simulink model "ddmr_for_mstc2003"  (R2022a)
settings: Solver=ode45  StartTime=0.0  StopTime=15  MaxStep=.1  MinStep=.001  RelTol=1e-3  EnableMultiTasking=on
libraries: dspsigattribs x28, matrix_library x6, dspinverses x3
settings Model: Creator=Orsted  LastModifiedBy=Orsted
settings SolverCC: InitialStep=.001
settings DataIOCC: LimitDataPoints=on  MaxDataPoints=10000  SaveFormat=Array  SignalLoggingSaveFormat=ModelDataLogs  ReturnWorkspaceOutputs=off  SignalLoggingName=sigsOut
settings OptimizationCC: BooleanDataType=off
settings DebuggingCC: SaveWithParameterizedLinksMsg=none  UnderspecifiedInitializationDetection=Classic  MergeDetectMultiDrivingBlocksExec=none  SignalResolutionControl=TryResolveAllWithWarning  MultiTaskDSMMsg=warning  MultiTaskCondExecSysMsg=none  UnconnectedInputMsg=warning  UnconnectedOutputMsg=warning  UnconnectedLineMsg=warning
settings HardwareCC: ProdBitPerPointer=32  ProdBitPerSizeT=32  ProdBitPerPtrDiffT=32  ProdLargestAtomicFloat=None  ProdIntDivRoundTo=Undefined  ProdEndianess=Unspecified  ProdWordSize=32  ProdHWDeviceType=32-bit Generic  TargetUnknown=on
settings ModelReferenceCC: PropagateSignalLabelsOutOfModel=off
settings GRTTargetCC: CombineOutputUpdateFcns=off  GRTInterface=on
settings ConfigComp: CovMetricSettings=dw  CovSaveCumulativeToWorkspaceVar=on  CovSaveSingleToWorkspaceVar=on

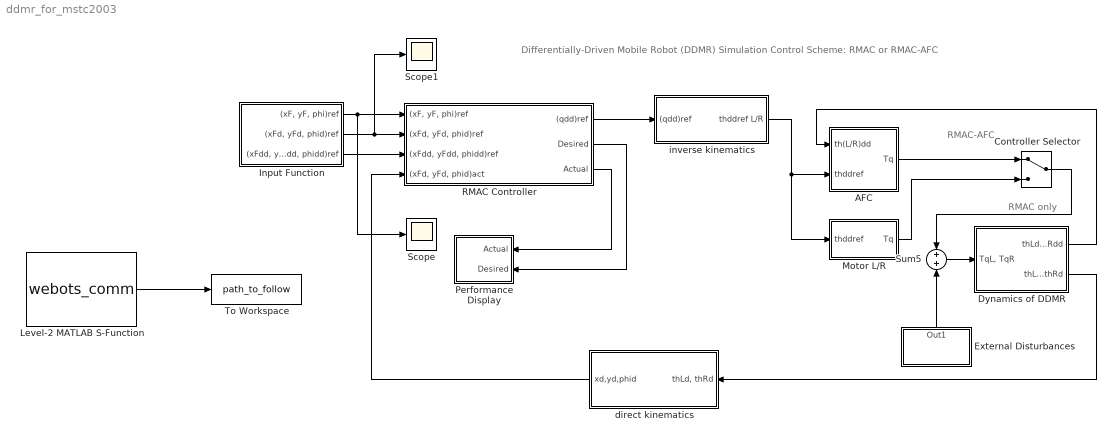
== system ddmr_for_mstc2003 ==
  note: Differentially-Driven Mobile Robot (DDMR) Simulation
      | Control Scheme: RMAC or RMAC-AFC
  note: RMAC-AFC
  note: RMAC only
  AFC : Subsystem  mask{IN=2.4, Ktn=.263}
      mask prompts: IN "Crude's Value (IN)"; Ktn "Motor Constant (Ktn)"
  Controller Selector : ManualSwitch
  Dynamics of DDMR : Subsystem  mask{phi=pi/2, d=.3, r=.11, mw=1, mc=40, b=.4, Ic=11.525, Im=.05, Iw=0.05}
      mask prompts: phi "Vehicle initial orientation (phi)"; d "Distance between Po to Pc (d)"; r "Radius of Wheels (r)"; mw "Mass of wheel (mw)"; mc "Mass of platform (mc)"; b "(1/2)Width of vehicle (b)"; Ic "Inertia of platform about vertical axis (Ic)"; Im "Inertia of wheel about wheel diameter (Im)"; Iw "Inertia of wheel about wheel axis (Iw)"
  External Disturbances : Subsystem  mask{Qtype=[5;6], Qc=[5;-5], Qpa=2, Qpf=1, Qsa=5, Qsf=5}
      mask prompts: Qtype "Disturbance Type: [1;2]Qconstant  [3;4]Qpulse  [5;6]Qsine"; Qc "Magnitude of Q-Constant (Qc)"; Qpa "Amplitude of Q-Pulse (Qpa)"; Qpf "Freq of Q-Pulse (Qpf)"; Qsa "Amplitude of Q-Sine (Qsa)"; Qsf "Freq of Q-Sine (Qsa)"
  Input Function : Subsystem  mask{phiref=pi/2, InSet=4, Vcut=.4, rinput=10}
      mask prompts: phiref "Vehicle Initial orientation (phiref)"; InSet "Input [ <1>Line-1 <2>Line-2 <3>Line-3 <4>Curve ]"; Vcut "Velocity of Running (Curve only)"; rinput "Radius of Curve"
  Level-2 MATLAB S-Function : M-S-Function  FunctionName=webots_comm
  Motor L/R : Subsystem
  Performance Display : Subsystem
  RMAC Controller : Subsystem  mask{qinit=[7;0;pi/2], Kp=[350;350;.005], Kd=[320;320;.0015]}
      mask prompts: qinit "Vehicle initial position (xF, yF, phi) > (qinit)"; Kp "Proportional Constant (Kp)"; Kd "Differential Constant (Kd)"
  Scope : Scope
  Scope1 : Scope
  Sum5 : Sum  InputSameDT=on  SaturateOnIntegerOverflow=on  OutDataTypeStr=Inherit: Same as first input
  To Workspace : ToWorkspace  VariableName=path_to_follow  SaveFormat=Structure With Time  SampleTime=-1
  direct kinematics : Subsystem  mask{phi=pi/2, b=0.4, r=0.11, lG=.3}
      mask prompts: phi "Vehicle initial orientation (phi)"; b "(1/2)Width of Body, b (m)"; r "Radius of wheels, r (m)"; lG "Distance between WG to WF (lG)"
  inverse kinematics : Subsystem  mask{phi=pi/2, b=0.4, r=0.11, lG=.3}
      mask prompts: phi "Vehicle initial orientation (phi)"; b "(1/2)Width of Body, b (m)"; r "Radius of wheels, r (m)"; lG "Distance between WG to WF (lG)"
  wires:
  Input Function/2("(xFd, yFd, phid)ref") -> Scope1/1, RMAC Controller/2("(xFd, yFd, phid)ref")
  RMAC Controller/1((qdd)ref) -> inverse kinematics/1((qdd)ref)
  Dynamics of DDMR/2("thLd, thRd") -> direct kinematics/1("thLd, thRd")
  Sum5/1 -> Dynamics of DDMR/1("TqL, TqR")
  Input Function/1("(xF, yF, phi)ref") -> Scope/1, RMAC Controller/1("(xF, yF, phi)ref")
  direct kinematics/1(xd,yd,phid) -> RMAC Controller/4("(xFd, yFd, phid)act")
  Input Function/3("(xFdd, yFdd, phidd)ref") -> RMAC Controller/3("(xFdd, yFdd, phidd)ref")
  External Disturbances/1(Out1) -> Sum5/2
  RMAC Controller/3(Actual) -> Performance Display/1(Actual)
  RMAC Controller/2(Desired) -> Performance Display/2(Desired)
  Dynamics of DDMR/1("thLdd, thRdd") -> AFC/1(th(L/R)dd)
  inverse kinematics/1(thddref L/R) -> AFC/2(thddref), Motor L/R/1(thddref)
  AFC/1(Tq) -> Controller Selector/1
  Controller Selector/1 -> Sum5/1
  Motor L/R/1(Tq) -> Controller Selector/2
  Level-2 MATLAB S-Function/1 -> To Workspace/1

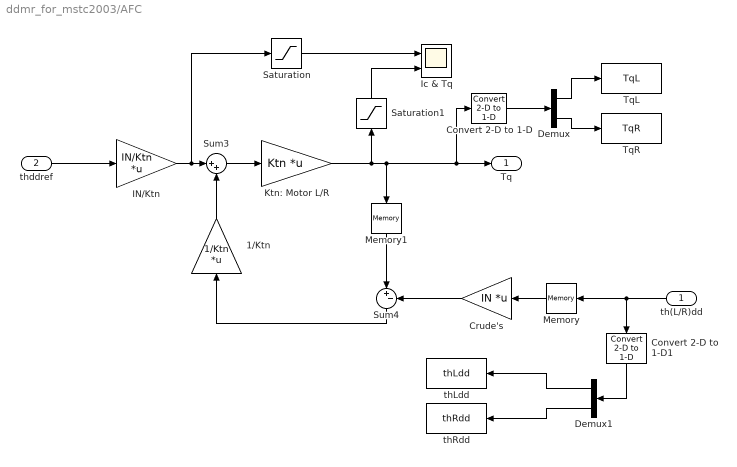
== system ddmr_for_mstc2003/AFC ==
  th(L/R)dd : Inport
  thddref : Inport  Port=2
  1/Ktn : Gain  Gain=1/Ktn  Multiplication=Matrix(K*u)  SaturateOnIntegerOverflow=on  OutDataTypeStr=Inherit: Same as input  ParamDataTypeStr=Inherit: Same as input
  Convert 2-D to 1-D : dspsigattribs/Convert 2-D to 1-D
      settings: SourceProductBaseCode=DS
  Convert 2-D to 1-D1 : dspsigattribs/Convert 2-D to 1-D
      settings: SourceProductBaseCode=DS
  Crude's : Gain  Gain=IN  Multiplication=Matrix(K*u)  SaturateOnIntegerOverflow=on  OutDataTypeStr=Inherit: Same as input  ParamDataTypeStr=Inherit: Same as input
  Demux : Demux  Outputs=2
      settings: DisplayOption=none
  Demux1 : Demux  Outputs=2
      settings: DisplayOption=none
  IN/Ktn : Gain  Gain=IN/Ktn  Multiplication=Matrix(K*u)  SaturateOnIntegerOverflow=on  OutDataTypeStr=Inherit: Same as input  ParamDataTypeStr=Inherit: Same as input
  Ic & Tq : Scope  NumInputPorts=2
  Ktn: Motor L/R : Gain  Gain=Ktn  Multiplication=Matrix(K*u)  SaturateOnIntegerOverflow=on  OutDataTypeStr=Inherit: Same as input  ParamDataTypeStr=Inherit: Same as input
  Memory : Memory
  Memory1 : Memory
  Saturation : Saturate  UpperLimit=30  LowerLimit=-30
  Saturation1 : Saturate  UpperLimit=30  LowerLimit=-30
  Sum3 : Sum  Inputs=|++  InputSameDT=on  SaturateOnIntegerOverflow=on  OutDataTypeStr=Inherit: Same as first input
  Sum4 : Sum  Inputs=|+-  InputSameDT=on  SaturateOnIntegerOverflow=on  OutDataTypeStr=Inherit: Same as first input
  TqL : ToWorkspace  VariableName=TqL  SampleTime=-1
  TqR : ToWorkspace  VariableName=TqR  SampleTime=-1
  thLdd : ToWorkspace  VariableName=thLdd  SampleTime=-1
  thRdd : ToWorkspace  VariableName=thRdd  SampleTime=-1
  Tq : Outport
  wires:
  Sum3/1 -> Ktn: Motor L/R/1
  IN/Ktn/1 -> Sum3/1, Saturation/1
  Crude's/1 -> Sum4/2
  Sum4/1 -> 1/Ktn/1
  1/Ktn/1 -> Sum3/2
  thddref/1 -> IN/Ktn/1
  th(L/R)dd/1 -> Memory/1, Convert 2-D to 1-D1/1
  Ktn: Motor L/R/1 -> Memory1/1, Tq/1, Convert 2-D to 1-D/1, Saturation1/1
  Saturation/1 -> Ic & Tq/1
  Saturation1/1 -> Ic & Tq/2
  Memory/1 -> Crude's/1
  Memory1/1 -> Sum4/1
  Demux/1 -> TqL/1
  Demux/2 -> TqR/1
  Convert 2-D to 1-D/1 -> Demux/1
  Demux1/1 -> thLdd/1
  Demux1/2 -> thRdd/1
  Convert 2-D to 1-D1/1 -> Demux1/1

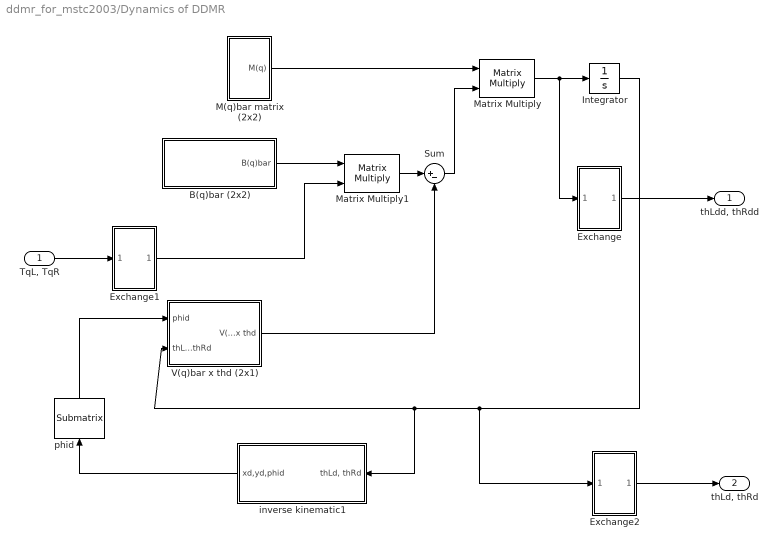
== system ddmr_for_mstc2003/Dynamics of DDMR ==
  "TqL, TqR" : Inport
  B(q)bar (2x2) : Subsystem
  Exchange : Subsystem
  Exchange1 : Subsystem
  Exchange2 : Subsystem
  Integrator : Integrator
  M(q)bar matrix (2x2) : Subsystem
  Matrix Multiply : Product  Multiplication=Matrix(*)
  Matrix Multiply1 : Product  Multiplication=Matrix(*)
  Sum : Sum  Inputs=|+-  InputSameDT=on  SaturateOnIntegerOverflow=on  OutDataTypeStr=Inherit: Same as first input
  V(q)bar x thd (2x1) : Subsystem
  inverse kinematic1 : Subsystem
  phid : matrix_library/Submatrix  RowSpan=Range of rows  RowStartMode=Index  RowStartIndex=3  RowEndMode=Last  RowEndIndex=1  ColSpan=Range of columns  ColStartMode=First  ColStartIndex=1  ColEndMode=Last  ColEndIndex=1
      settings: SourceProductBaseCode=SL
  "thLdd, thRdd" : Outport
  "thLd, thRd" : Outport  Port=2
  wires:
  M(q)bar matrix (2x2)/1(M(q)) -> Matrix Multiply/1
  B(q)bar (2x2)/1(B(q)bar) -> Matrix Multiply1/1
  "TqL, TqR"/1 -> Exchange1/1(In1)
  Matrix Multiply1/1 -> Sum/1
  V(q)bar x thd (2x1)/1(V(q) bar x thd) -> Sum/2
  Sum/1 -> Matrix Multiply/2
  Matrix Multiply/1 -> Integrator/1, Exchange/1(In1)
  Integrator/1 -> V(q)bar x thd (2x1)/2("thLd, thRd"), inverse kinematic1/1("thLd, thRd"), Exchange2/1(In1)
  inverse kinematic1/1(xd,yd,phid) -> phid/1
  phid/1 -> V(q)bar x thd (2x1)/1(phid)
  Exchange2/1(Out1) -> "thLd, thRd"/1
  Exchange1/1(Out1) -> Matrix Multiply1/2
  Exchange/1(Out1) -> "thLdd, thRdd"/1

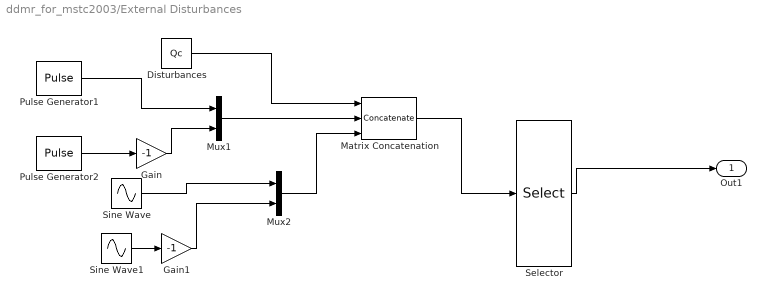
== system ddmr_for_mstc2003/External Disturbances ==
  Disturbances : Constant  Value=Qc  VectorParams1D=off
  Gain : Gain  Gain=-1  SaturateOnIntegerOverflow=on  OutDataTypeStr=Inherit: Same as input  ParamDataTypeStr=Inherit: Same as input
  Gain1 : Gain  Gain=-1  SaturateOnIntegerOverflow=on  OutDataTypeStr=Inherit: Same as input  ParamDataTypeStr=Inherit: Same as input
  Matrix Concatenation : Concatenate  NumInputs=3  Mode=Multidimensional array
  Mux1 : Mux  Inputs=2
  Mux2 : Mux  Inputs=2
  Pulse Generator1 : DiscretePulseGenerator  PulseType=Time based  Amplitude=Qpa  Period=Qpf  PulseWidth=50
  Pulse Generator2 : DiscretePulseGenerator  PulseType=Time based  Amplitude=Qpa  Period=Qpf  PulseWidth=50
  Selector : Selector  InputPortWidth=6  IndexOptions=Index vector (dialog)  Indices=Qtype  OutputSizes=1
  Sine Wave : Sin  Amplitude=Qsa  Frequency=Qsf  SampleTime=0
  Sine Wave1 : Sin  Amplitude=Qsa  Frequency=Qsf  SampleTime=0
  Out1 : Outport
  wires:
  Selector/1 -> Out1/1
  Pulse Generator1/1 -> Mux1/1
  Pulse Generator2/1 -> Gain/1
  Sine Wave/1 -> Mux2/1
  Sine Wave1/1 -> Gain1/1
  Disturbances/1 -> Matrix Concatenation/1
  Mux1/1 -> Matrix Concatenation/2
  Mux2/1 -> Matrix Concatenation/3
  Matrix Concatenation/1 -> Selector/1
  Gain/1 -> Mux1/2
  Gain1/1 -> Mux2/2

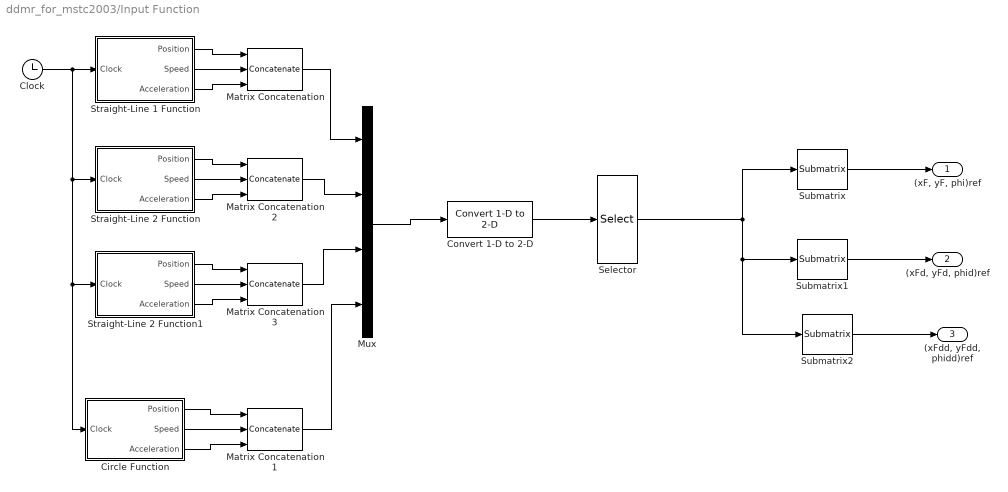
== system ddmr_for_mstc2003/Input Function ==
  Circle Function : Subsystem
  Clock : Clock
  Convert 1-D to 2-D : dspsigattribs/Convert 1-D to 2-D  M=9  N=4  frameBasedOut=off
      settings: SourceProductBaseCode=DS
  Matrix Concatenation{,1..3} (4 alike) : Concatenate  NumInputs=3  Mode=Multidimensional array
  Mux : Mux
  Selector : Selector  NumberOfDimensions=2  InputPortWidth=2  IndexOptions=Select all,Index vector (dialog)  Indices=-1,InSet  OutputSizes=1,
  Straight-Line 1 Function : Subsystem
  Straight-Line 2 Function : Subsystem
  Straight-Line 2 Function1 : Subsystem
  Submatrix : matrix_library/Submatrix  RowSpan=Range of rows  RowStartMode=First  RowStartIndex=1  RowEndMode=Index  RowEndIndex=3  ColSpan=Range of columns  ColStartMode=First  ColStartIndex=1  ColEndMode=Last  ColEndIndex=1
      settings: SourceProductBaseCode=SL
  Submatrix1 : matrix_library/Submatrix  RowSpan=Range of rows  RowStartMode=Index  RowStartIndex=4  RowEndMode=Index  RowEndIndex=6  ColSpan=Range of columns  ColStartMode=First  ColStartIndex=1  ColEndMode=Last  ColEndIndex=1
      settings: SourceProductBaseCode=SL
  Submatrix2 : matrix_library/Submatrix  RowSpan=Range of rows  RowStartMode=Index  RowStartIndex=7  RowEndMode=Index  RowEndIndex=9  ColSpan=Range of columns  ColStartMode=First  ColStartIndex=1  ColEndMode=Last  ColEndIndex=1
      settings: SourceProductBaseCode=SL
  "(xF, yF, phi)ref" : Outport
  "(xFd, yFd, phid)ref" : Outport  Port=2
  "(xFdd, yFdd, phidd)ref" : Outport  Port=3
  wires:
  Clock/1 -> Straight-Line 1 Function/1(Clock), Straight-Line 2 Function/1(Clock), Circle Function/1(Clock), Straight-Line 2 Function1/1(Clock)
  Straight-Line 1 Function/1(Position) -> Matrix Concatenation/1
  Straight-Line 1 Function/2(Speed) -> Matrix Concatenation/2
  Straight-Line 1 Function/3(Acceleration) -> Matrix Concatenation/3
  Circle Function/1(Position) -> Matrix Concatenation1/1
  Circle Function/2(Speed) -> Matrix Concatenation1/2
  Circle Function/3(Acceleration) -> Matrix Concatenation1/3
  Selector/1 -> Submatrix1/1, Submatrix2/1, Submatrix/1
  Matrix Concatenation/1 -> Mux/1
  Submatrix/1 -> "(xF, yF, phi)ref"/1
  Submatrix1/1 -> "(xFd, yFd, phid)ref"/1
  Submatrix2/1 -> "(xFdd, yFdd, phidd)ref"/1
  Mux/1 -> Convert 1-D to 2-D/1
  Convert 1-D to 2-D/1 -> Selector/1
  Straight-Line 2 Function/1(Position) -> Matrix Concatenation2/1
  Straight-Line 2 Function/2(Speed) -> Matrix Concatenation2/2
  Straight-Line 2 Function/3(Acceleration) -> Matrix Concatenation2/3
  Matrix Concatenation2/1 -> Mux/2
  Straight-Line 2 Function1/1(Position) -> Matrix Concatenation3/1
  Straight-Line 2 Function1/2(Speed) -> Matrix Concatenation3/2
  Straight-Line 2 Function1/3(Acceleration) -> Matrix Concatenation3/3
  Matrix Concatenation3/1 -> Mux/3
  Matrix Concatenation1/1 -> Mux/4

== system ddmr_for_mstc2003/Motor L//R ==
  thddref : Inport
  Convert 2-D to 1-D : dspsigattribs/Convert 2-D to 1-D
      settings: SourceProductBaseCode=DS
  Demux : Demux  Outputs=2
      settings: DisplayOption=none
  Motor L/R : Gain  Gain=.263  SaturateOnIntegerOverflow=on  OutDataTypeStr=Inherit: Same as input  ParamDataTypeStr=Inherit: Same as input
  To Workspace : ToWorkspace  VariableName=TqLpd  SampleTime=-1
  To Workspace1 : ToWorkspace  VariableName=TqRpd  SampleTime=-1
  Tq : Outport
  wires:
  thddref/1 -> Motor L/R/1
  Motor L/R/1 -> Tq/1, Convert 2-D to 1-D/1
  Convert 2-D to 1-D/1 -> Demux/1
  Demux/1 -> To Workspace/1
  Demux/2 -> To Workspace1/1

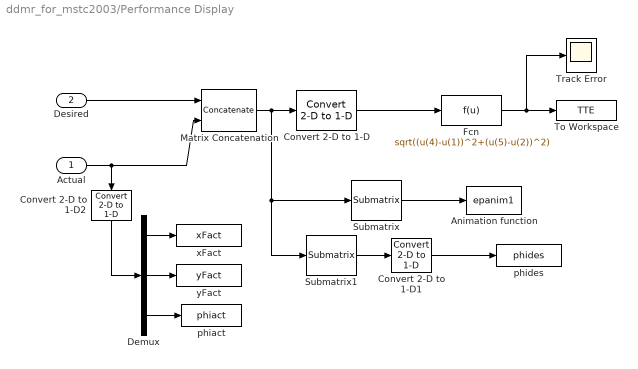
== system ddmr_for_mstc2003/Performance Display ==
  Actual : Inport
  Desired : Inport  Port=2
  Animation function : S-Function  FunctionName=epanim1  Parameters=.1  SFunctionDeploymentMode=off  EnableBusSupport=off
      settings: DeleteFcn=if ~isempty(findobj('type','figure','name','onecart Animation'));close('onecart Animation'); end;
  Convert 2-D to 1-D : dspsigattribs/Convert 2-D to 1-D
      settings: SourceProductBaseCode=DS
  Convert 2-D to 1-D1 : dspsigattribs/Convert 2-D to 1-D
      settings: SourceProductBaseCode=DS
  Convert 2-D to 1-D2 : dspsigattribs/Convert 2-D to 1-D
      settings: SourceProductBaseCode=DS
  Demux : Demux  Outputs=3
      settings: DisplayOption=none
  Fcn : Fcn  Expr=sqrt((u(4)-u(1))^2+(u(5)-u(2))^2)
  Matrix Concatenation : Concatenate  Mode=Multidimensional array
  Submatrix : matrix_library/Submatrix  RowSpan=Range of rows  RowStartMode=Index  RowStartIndex=4  RowEndMode=Index  RowEndIndex=6  ColSpan=Range of columns  ColStartMode=First  ColStartIndex=1  ColEndMode=Last  ColEndIndex=1
      settings: SourceProductBaseCode=SL
  Submatrix1 : matrix_library/Submatrix  RowSpan=Range of rows  RowStartMode=Index  RowStartIndex=3  RowEndMode=Index  RowEndIndex=3  ColSpan=Range of columns  ColStartMode=First  ColStartIndex=1  ColEndMode=Last  ColEndIndex=1
      settings: SourceProductBaseCode=SL
  To Workspace : ToWorkspace  VariableName=TTE  SampleTime=-1
  Track Error : Scope
  phiact : ToWorkspace  VariableName=phiact  SampleTime=-1
  phides : ToWorkspace  VariableName=phides  SampleTime=-1
  xFact : ToWorkspace  VariableName=xFact  SampleTime=-1
  yFact : ToWorkspace  VariableName=yFact  SampleTime=-1
  wires:
  Actual/1 -> Matrix Concatenation/2, Convert 2-D to 1-D2/1
  Matrix Concatenation/1 -> Convert 2-D to 1-D/1, Submatrix/1, Submatrix1/1
  Convert 2-D to 1-D/1 -> Fcn/1
  Desired/1 -> Matrix Concatenation/1
  Fcn/1 -> To Workspace/1, Track Error/1
  Submatrix/1 -> Animation function/1
  Submatrix1/1 -> Convert 2-D to 1-D1/1
  Convert 2-D to 1-D1/1 -> phides/1
  Demux/1 -> xFact/1
  Demux/2 -> yFact/1
  Demux/3 -> phiact/1
  Convert 2-D to 1-D2/1 -> Demux/1

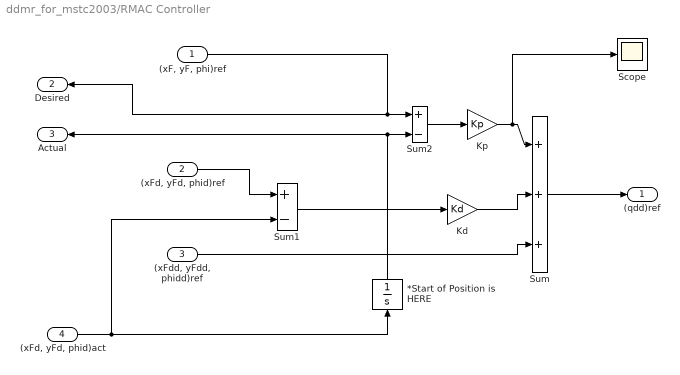
== system ddmr_for_mstc2003/RMAC Controller ==
  "(xF, yF, phi)ref" : Inport
  "(xFd, yFd, phid)ref" : Inport  Port=2
  "(xFdd, yFdd, phidd)ref" : Inport  Port=3
  "(xFd, yFd, phid)act" : Inport  Port=4
  *Start of Position is HERE : Integrator  InitialCondition=qinit
  "Kd " : Gain  Gain=Kd  SaturateOnIntegerOverflow=on  OutDataTypeStr=Inherit: Same as input  ParamDataTypeStr=Inherit: Same as input
  Kp : Gain  Gain=Kp  SaturateOnIntegerOverflow=on  OutDataTypeStr=Inherit: Same as input  ParamDataTypeStr=Inherit: Same as input
  Scope : Scope
  Sum : Sum  Inputs=+++  InputSameDT=on  SaturateOnIntegerOverflow=on  OutDataTypeStr=Inherit: Same as first input
  Sum1 : Sum  Inputs=+-  InputSameDT=on  SaturateOnIntegerOverflow=on  OutDataTypeStr=Inherit: Same as first input
  Sum2 : Sum  Inputs=+-  InputSameDT=on  SaturateOnIntegerOverflow=on  OutDataTypeStr=Inherit: Same as first input
  (qdd)ref : Outport
  Desired : Outport  Port=2
  Actual : Outport  Port=3
  wires:
  Sum1/1 -> "Kd "/1
  Sum2/1 -> Kp/1
  "Kd "/1 -> Sum/2
  Kp/1 -> Sum/1, Scope/1
  *Start of Position is HERE/1 -> Sum2/2, Actual/1
  "(xF, yF, phi)ref"/1 -> Sum2/1, Desired/1
  Sum/1 -> (qdd)ref/1
  "(xFd, yFd, phid)ref"/1 -> Sum1/1
  "(xFd, yFd, phid)act"/1 -> *Start of Position is HERE/1, Sum1/2
  "(xFdd, yFdd, phidd)ref"/1 -> Sum/3

== system ddmr_for_mstc2003/direct kinematics ==
  "thLd, thRd" : Inport
  Exchange1 : Subsystem
  Integrator : Integrator  InitialCondition=phi
  Matrix Multiply : Product  Multiplication=Matrix(*)
  S*(q) matrix (3x2) : Subsystem
  To Workspace : ToWorkspace  VariableName=idksfterexc  SaveFormat=Structure With Time  SampleTime=-1
  xd,yd,phid : Outport
  wires:
  "thLd, thRd"/1 -> Exchange1/1(In1)
  Matrix Multiply/1 -> xd,yd,phid/1, Integrator/1
  Integrator/1 -> S*(q) matrix (3x2)/1(phi)
  Exchange1/1(Out1) -> To Workspace/1, Matrix Multiply/2
  S*(q) matrix (3x2)/1(S*(q)) -> Matrix Multiply/1

== system ddmr_for_mstc2003/inverse kinematics ==
  (qdd)ref : Inport
  Convert 1-D to 2-D : dspsigattribs/Convert 1-D to 2-D  M=3  N=1  frameBasedOut=off
      settings: SourceProductBaseCode=DS
  Exchange1 : Subsystem
  Integrator : Integrator  InitialCondition=phi
  Matrix Multiply : Product  Multiplication=Matrix(*)
  Pseudoinverse : dspinverses/Pseudoinverse  wanterr=off  SimulateUsing=Interpreted execution
      settings: SourceProductBaseCode=DS
  S*(q) matrix (3x2) : Subsystem
  thddref L/R : Outport
  wires:
  Pseudoinverse/1 -> Matrix Multiply/1
  (qdd)ref/1 -> Convert 1-D to 2-D/1, Integrator/1
  Matrix Multiply/1 -> Exchange1/1(In1)
  Convert 1-D to 2-D/1 -> Matrix Multiply/2
  Integrator/1 -> S*(q) matrix (3x2)/1(phi)
  S*(q) matrix (3x2)/1(S*(q)) -> Pseudoinverse/1
  Exchange1/1(Out1) -> thddref L/R/1

== system ddmr_for_mstc2003/Dynamics of DDMR/B(q)bar (2x2) ==
  Constant1 : Constant  Value=0
  Constant2 : Constant
  Constant3 : Constant  Value=0
  Constant4 : Constant
  Convert 1-D to 2-D : dspsigattribs/Convert 1-D to 2-D  M=2  N=2  frameBasedOut=off
      settings: SourceProductBaseCode=DS
  Mux : Mux
  B(q)bar : Outport
  wires:
  Mux/1 -> Convert 1-D to 2-D/1
  Constant2/1 -> Mux/1
  Constant1/1 -> Mux/2
  Constant3/1 -> Mux/3
  Constant4/1 -> Mux/4
  Convert 1-D to 2-D/1 -> B(q)bar/1

== system ddmr_for_mstc2003/Dynamics of DDMR/Exchange ==
  In1 : Inport
  Convert 1-D to 2-D2 : dspsigattribs/Convert 1-D to 2-D  M=2  N=1  frameBasedOut=off
      settings: SourceProductBaseCode=DS
  Convert 2-D to 1-D2 : dspsigattribs/Convert 2-D to 1-D
      settings: SourceProductBaseCode=DS
  Demux2 : Demux  Outputs=2
      settings: DisplayOption=none
  Mux2 : Mux  Inputs=2
  Out1 : Outport
  wires:
  Mux2/1 -> Convert 1-D to 2-D2/1
  Demux2/1 -> Mux2/2
  Demux2/2 -> Mux2/1
  Convert 2-D to 1-D2/1 -> Demux2/1
  In1/1 -> Convert 2-D to 1-D2/1
  Convert 1-D to 2-D2/1 -> Out1/1

== system ddmr_for_mstc2003/Dynamics of DDMR/Exchange1 ==
  In1 : Inport
  Convert 1-D to 2-D2 : dspsigattribs/Convert 1-D to 2-D  M=2  N=1  frameBasedOut=off
      settings: SourceProductBaseCode=DS
  Convert 2-D to 1-D2 : dspsigattribs/Convert 2-D to 1-D
      settings: SourceProductBaseCode=DS
  Demux2 : Demux  Outputs=2
      settings: DisplayOption=none
  Mux2 : Mux  Inputs=2
  Out1 : Outport
  wires:
  Mux2/1 -> Convert 1-D to 2-D2/1
  Demux2/1 -> Mux2/2
  Demux2/2 -> Mux2/1
  Convert 2-D to 1-D2/1 -> Demux2/1
  In1/1 -> Convert 2-D to 1-D2/1
  Convert 1-D to 2-D2/1 -> Out1/1

== system ddmr_for_mstc2003/Dynamics of DDMR/Exchange2 ==
  In1 : Inport
  Convert 1-D to 2-D2 : dspsigattribs/Convert 1-D to 2-D  M=2  N=1  frameBasedOut=off
      settings: SourceProductBaseCode=DS
  Convert 2-D to 1-D2 : dspsigattribs/Convert 2-D to 1-D
      settings: SourceProductBaseCode=DS
  Demux2 : Demux  Outputs=2
      settings: DisplayOption=none
  Mux2 : Mux  Inputs=2
  Out1 : Outport
  wires:
  Mux2/1 -> Convert 1-D to 2-D2/1
  Demux2/1 -> Mux2/2
  Demux2/2 -> Mux2/1
  Convert 2-D to 1-D2/1 -> Demux2/1
  In1/1 -> Convert 2-D to 1-D2/1
  Convert 1-D to 2-D2/1 -> Out1/1

== system ddmr_for_mstc2003/Dynamics of DDMR/M(q)bar matrix (2x2) ==
  Convert 1-D to 2-D : dspsigattribs/Convert 1-D to 2-D  M=2  N=2  frameBasedOut=off
      settings: SourceProductBaseCode=DS
  M11 : Constant  Value=(r^2)/(4*(b^2))*((mc+2*mw)*(b^2)+(mc*(d^2)+2*mw*(b^2)+Ic+2*Im))+Iw
  M12 : Constant  Value=(r^2)/(4*(b^2))*((mc+2*mw)*(b^2)-(mc*(d^2)+2*mw*(b^2)+Ic+2*Im))
  M21 : Constant  Value=(r^2)/(4*(b^2))*((mc+2*mw)*(b^2)-(mc*(d^2)+2*mw*(b^2)+Ic+2*Im))
  M22 : Constant  Value=(r^2)/(4*(b^2))*((mc+2*mw)*(b^2)+(mc*(d^2)+2*mw*(b^2)+Ic+2*Im))+Iw
  Mux : Mux
  M(q) : Outport
  wires:
  M11/1 -> Mux/1
  M12/1 -> Mux/2
  M21/1 -> Mux/3
  M22/1 -> Mux/4
  Mux/1 -> Convert 1-D to 2-D/1
  Convert 1-D to 2-D/1 -> M(q)/1

== system ddmr_for_mstc2003/Dynamics of DDMR/V(q)bar x thd (2x1) ==
  phid : Inport
  "thLd, thRd" : Inport  Port=2
  Matrix Multiply3 : Product  Multiplication=Matrix(*)
  V(q,qd)bar (3x1) : Subsystem
  V(q) bar x thd : Outport
  wires:
  Matrix Multiply3/1 -> V(q) bar x thd/1
  V(q,qd)bar (3x1)/1(V(q,qd)bar) -> Matrix Multiply3/1
  phid/1 -> V(q,qd)bar (3x1)/1(phid)
  "thLd, thRd"/1 -> Matrix Multiply3/2

== system ddmr_for_mstc2003/Dynamics of DDMR/inverse kinematic1 ==
  "thLd, thRd" : Inport
  Convert 1-D to 2-D : dspsigattribs/Convert 1-D to 2-D  M=2  N=1  frameBasedOut=off
      settings: SourceProductBaseCode=DS
  Convert 2-D to 1-D : dspsigattribs/Convert 2-D to 1-D
      settings: SourceProductBaseCode=DS
  Demux : Demux  Outputs=2
      settings: DisplayOption=none
  Integrator : Integrator  InitialCondition=phi
  Matrix Multiply : Product  Multiplication=Matrix(*)
  Mux : Mux  Inputs=2
  S(q) matrix (3x2) : Subsystem
  xd,yd,phid : Outport
  wires:
  S(q) matrix (3x2)/1(S(q)) -> Matrix Multiply/1
  Matrix Multiply/1 -> xd,yd,phid/1, Integrator/1
  Integrator/1 -> S(q) matrix (3x2)/1(phi)
  Mux/1 -> Convert 1-D to 2-D/1
  Demux/1 -> Mux/2
  Demux/2 -> Mux/1
  Convert 2-D to 1-D/1 -> Demux/1
  Convert 1-D to 2-D/1 -> Matrix Multiply/2
  "thLd, thRd"/1 -> Convert 2-D to 1-D/1

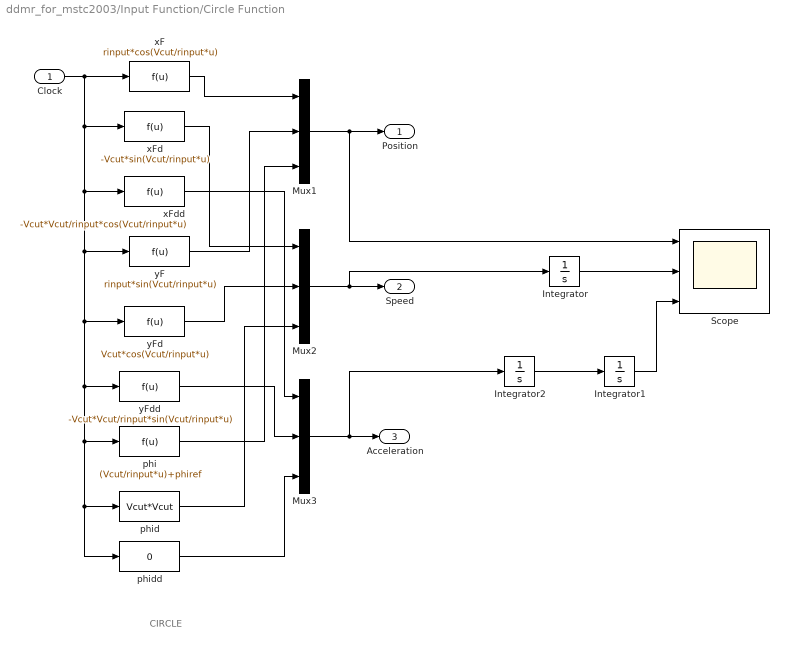
== system ddmr_for_mstc2003/Input Function/Circle Function ==
  note: CIRCLE
  Clock : Inport
  Integrator : Integrator  InitialCondition=[10;0;pi/2]
  Integrator1 : Integrator  InitialCondition=[10;0;pi/2]
  Integrator2 : Integrator  InitialCondition=[0;Vcut;Vcut*Vcut]
  Mux1 : Mux  Inputs=3
  Mux2 : Mux  Inputs=3
  Mux3 : Mux  Inputs=3
  Scope : Scope  NumInputPorts=3
  phi : Fcn  Expr=(Vcut/rinput*u)+phiref
  phid : Fcn  Expr=Vcut*Vcut
  phidd : Fcn  Expr=0
  xF : Fcn  Expr=rinput*cos(Vcut/rinput*u)
  xFd : Fcn  Expr=-Vcut*sin(Vcut/rinput*u)
  xFdd : Fcn  Expr=-Vcut*Vcut/rinput*cos(Vcut/rinput*u)
  yF : Fcn  Expr=rinput*sin(Vcut/rinput*u)
  yFd : Fcn  Expr=Vcut*cos(Vcut/rinput*u)
  yFdd : Fcn  Expr=-Vcut*Vcut/rinput*sin(Vcut/rinput*u)
  Position : Outport
  Speed : Outport  Port=2
  Acceleration : Outport  Port=3
  wires:
  Clock/1 -> xF/1, xFd/1, xFdd/1, yF/1, phidd/1, phid/1, phi/1, yFdd/1, yFd/1
  yF/1 -> Mux1/2
  yFd/1 -> Mux2/2
  xFd/1 -> Mux2/1
  xF/1 -> Mux1/1
  phi/1 -> Mux1/3
  phid/1 -> Mux2/3
  xFdd/1 -> Mux3/1
  yFdd/1 -> Mux3/2
  phidd/1 -> Mux3/3
  Mux1/1 -> Position/1, Scope/1
  Mux2/1 -> Speed/1, Integrator/1
  Mux3/1 -> Acceleration/1, Integrator2/1
  Integrator/1 -> Scope/2
  Integrator1/1 -> Scope/3
  Integrator2/1 -> Integrator1/1

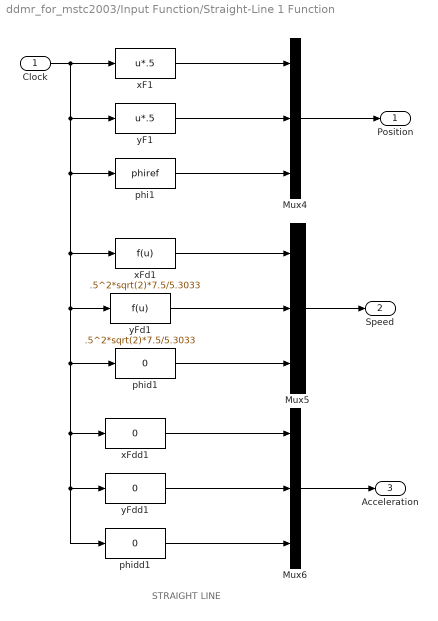
== system ddmr_for_mstc2003/Input Function/Straight-Line 1 Function ==
  note: STRAIGHT LINE
  Clock : Inport
  Mux4 : Mux  Inputs=3
  Mux5 : Mux  Inputs=3
  Mux6 : Mux  Inputs=3
  phi1 : Fcn  Expr=phiref
  phid1 : Fcn  Expr=0
  phidd1 : Fcn  Expr=0
  xF1 : Fcn  Expr=u*.5
  xFd1 : Fcn  Expr=.5^2*sqrt(2)*7.5/5.3033
  xFdd1 : Fcn  Expr=0
  yF1 : Fcn  Expr=u*.5
  yFd1 : Fcn  Expr=.5^2*sqrt(2)*7.5/5.3033
  yFdd1 : Fcn  Expr=0
  Position : Outport
  Speed : Outport  Port=2
  Acceleration : Outport  Port=3
  wires:
  Clock/1 -> xF1/1, phi1/1, yFd1/1, phidd1/1, yFdd1/1, xFdd1/1, phid1/1, xFd1/1, yF1/1
  Mux4/1 -> Position/1
  Mux5/1 -> Speed/1
  Mux6/1 -> Acceleration/1
  xF1/1 -> Mux4/1
  phi1/1 -> Mux4/3
  yFd1/1 -> Mux5/2
  phid1/1 -> Mux5/3
  xFdd1/1 -> Mux6/1
  yFdd1/1 -> Mux6/2
  phidd1/1 -> Mux6/3
  yF1/1 -> Mux4/2
  xFd1/1 -> Mux5/1

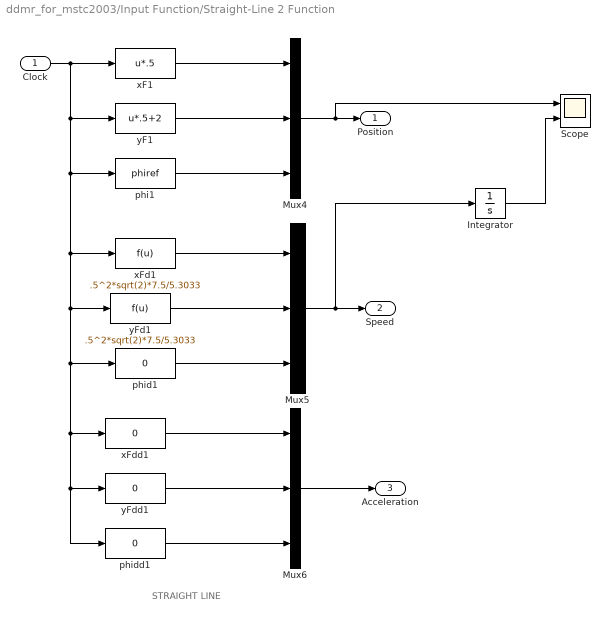
== system ddmr_for_mstc2003/Input Function/Straight-Line 2 Function ==
  note: STRAIGHT LINE
  Clock : Inport
  Integrator : Integrator  InitialCondition=[-2;2;pi/4]
  Mux4 : Mux  Inputs=3
  Mux5 : Mux  Inputs=3
  Mux6 : Mux  Inputs=3
  Scope : Scope  NumInputPorts=2
  phi1 : Fcn  Expr=phiref
  phid1 : Fcn  Expr=0
  phidd1 : Fcn  Expr=0
  xF1 : Fcn  Expr=u*.5
  xFd1 : Fcn  Expr=.5^2*sqrt(2)*7.5/5.3033
  xFdd1 : Fcn  Expr=0
  yF1 : Fcn  Expr=u*.5+2
  yFd1 : Fcn  Expr=.5^2*sqrt(2)*7.5/5.3033
  yFdd1 : Fcn  Expr=0
  Position : Outport
  Speed : Outport  Port=2
  Acceleration : Outport  Port=3
  wires:
  Clock/1 -> xF1/1, phi1/1, yFd1/1, phidd1/1, yFdd1/1, xFdd1/1, phid1/1, xFd1/1, yF1/1
  Mux4/1 -> Position/1, Scope/1
  Mux5/1 -> Speed/1, Integrator/1
  Mux6/1 -> Acceleration/1
  xF1/1 -> Mux4/1
  phi1/1 -> Mux4/3
  yFd1/1 -> Mux5/2
  phid1/1 -> Mux5/3
  xFdd1/1 -> Mux6/1
  yFdd1/1 -> Mux6/2
  phidd1/1 -> Mux6/3
  yF1/1 -> Mux4/2
  xFd1/1 -> Mux5/1
  Integrator/1 -> Scope/2

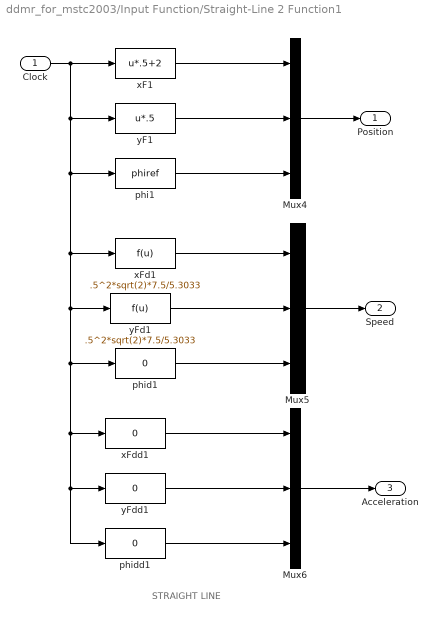
== system ddmr_for_mstc2003/Input Function/Straight-Line 2 Function1 ==
  note: STRAIGHT LINE
  Clock : Inport
  Mux4 : Mux  Inputs=3
  Mux5 : Mux  Inputs=3
  Mux6 : Mux  Inputs=3
  phi1 : Fcn  Expr=phiref
  phid1 : Fcn  Expr=0
  phidd1 : Fcn  Expr=0
  xF1 : Fcn  Expr=u*.5+2
  xFd1 : Fcn  Expr=.5^2*sqrt(2)*7.5/5.3033
  xFdd1 : Fcn  Expr=0
  yF1 : Fcn  Expr=u*.5
  yFd1 : Fcn  Expr=.5^2*sqrt(2)*7.5/5.3033
  yFdd1 : Fcn  Expr=0
  Position : Outport
  Speed : Outport  Port=2
  Acceleration : Outport  Port=3
  wires:
  Clock/1 -> xF1/1, phi1/1, yFd1/1, phidd1/1, yFdd1/1, xFdd1/1, phid1/1, xFd1/1, yF1/1
  Mux4/1 -> Position/1
  Mux5/1 -> Speed/1
  Mux6/1 -> Acceleration/1
  xF1/1 -> Mux4/1
  phi1/1 -> Mux4/3
  yFd1/1 -> Mux5/2
  phid1/1 -> Mux5/3
  xFdd1/1 -> Mux6/1
  yFdd1/1 -> Mux6/2
  phidd1/1 -> Mux6/3
  yF1/1 -> Mux4/2
  xFd1/1 -> Mux5/1

== system ddmr_for_mstc2003/direct kinematics/Exchange1 ==
  In1 : Inport
  Convert 1-D to 2-D2 : dspsigattribs/Convert 1-D to 2-D  M=2  N=1  frameBasedOut=off
      settings: SourceProductBaseCode=DS
  Convert 2-D to 1-D2 : dspsigattribs/Convert 2-D to 1-D
      settings: SourceProductBaseCode=DS
  Demux2 : Demux  Outputs=2
      settings: DisplayOption=none
  Mux2 : Mux  Inputs=2
  Out1 : Outport
  wires:
  Mux2/1 -> Convert 1-D to 2-D2/1
  Demux2/1 -> Mux2/2
  Demux2/2 -> Mux2/1
  Convert 2-D to 1-D2/1 -> Demux2/1
  In1/1 -> Convert 2-D to 1-D2/1
  Convert 1-D to 2-D2/1 -> Out1/1

== system ddmr_for_mstc2003/direct kinematics/S*(q) matrix (3x2) ==
  phi : Inport
  Matrix Multiply1 : Product  Multiplication=Matrix(*)
  Pseudoinverse1 : dspinverses/Pseudoinverse  wanterr=off  SimulateUsing=Interpreted execution
      settings: SourceProductBaseCode=DS
  S(q) matrix (3x2)1 : Subsystem
  Subsystem : Subsystem
  S*(q) : Outport
  wires:
  S(q) matrix (3x2)1/1(S(q)) -> Matrix Multiply1/1
  Subsystem/1(br(q)) -> Pseudoinverse1/1
  Pseudoinverse1/1 -> Matrix Multiply1/2
  phi/1 -> S(q) matrix (3x2)1/1(phi)
  Matrix Multiply1/1 -> S*(q)/1

== system ddmr_for_mstc2003/inverse kinematics/Exchange1 ==
  In1 : Inport
  Convert 1-D to 2-D2 : dspsigattribs/Convert 1-D to 2-D  M=2  N=1  frameBasedOut=off
      settings: SourceProductBaseCode=DS
  Convert 2-D to 1-D2 : dspsigattribs/Convert 2-D to 1-D
      settings: SourceProductBaseCode=DS
  Demux2 : Demux  Outputs=2
      settings: DisplayOption=none
  Mux2 : Mux  Inputs=2
  Out1 : Outport
  wires:
  Mux2/1 -> Convert 1-D to 2-D2/1
  Demux2/1 -> Mux2/2
  Demux2/2 -> Mux2/1
  Convert 2-D to 1-D2/1 -> Demux2/1
  In1/1 -> Convert 2-D to 1-D2/1
  Convert 1-D to 2-D2/1 -> Out1/1

== system ddmr_for_mstc2003/inverse kinematics/S*(q) matrix (3x2) ==
  phi : Inport
  Matrix Multiply1 : Product  Multiplication=Matrix(*)
  Pseudoinverse1 : dspinverses/Pseudoinverse  wanterr=off  SimulateUsing=Interpreted execution
      settings: SourceProductBaseCode=DS
  S(q) matrix (3x2)1 : Subsystem
  Subsystem : Subsystem
  S*(q) : Outport
  wires:
  S(q) matrix (3x2)1/1(S(q)) -> Matrix Multiply1/1
  Subsystem/1(br(q)) -> Pseudoinverse1/1
  Pseudoinverse1/1 -> Matrix Multiply1/2
  phi/1 -> S(q) matrix (3x2)1/1(phi)
  Matrix Multiply1/1 -> S*(q)/1

== system ddmr_for_mstc2003/Dynamics of DDMR/V(q)bar x thd (2x1)/V(q,qd)bar (3x1) ==
  phid : Inport
  Constant1 : Constant  Value=0
  Constant2 : Constant  Value=0
  Convert 1-D to 2-D : dspsigattribs/Convert 1-D to 2-D  M=2  N=2  frameBasedOut=off
      settings: SourceProductBaseCode=DS
  Fcn2 : Fcn  Expr=-(r^2)/2*b*mc*d*u
  Fcn3 : Fcn  Expr=(r^2)/2*b*mc*d*u
  Mux : Mux
  V(q,qd)bar : Outport
  wires:
  Convert 1-D to 2-D/1 -> V(q,qd)bar/1
  Mux/1 -> Convert 1-D to 2-D/1
  Constant2/1 -> Mux/1
  Fcn2/1 -> Mux/2
  Fcn3/1 -> Mux/3
  Constant1/1 -> Mux/4
  phid/1 -> Fcn2/1, Fcn3/1

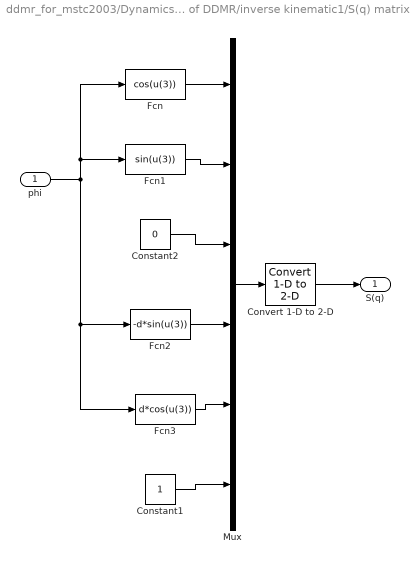
== system ddmr_for_mstc2003/Dynamics of DDMR/inverse kinematic1/S(q) matrix (3x2) ==
  phi : Inport
  Constant1 : Constant
  Constant2 : Constant  Value=0
  Convert 1-D to 2-D : dspsigattribs/Convert 1-D to 2-D  M=3  N=2  frameBasedOut=off
      settings: SourceProductBaseCode=DS
  Fcn : Fcn  Expr=cos(u(3))
  Fcn1 : Fcn  Expr=sin(u(3))
  Fcn2 : Fcn  Expr=-d*sin(u(3))
  Fcn3 : Fcn  Expr=d*cos(u(3))
  Mux : Mux  Inputs=6
  S(q) : Outport
  wires:
  Mux/1 -> Convert 1-D to 2-D/1
  Convert 1-D to 2-D/1 -> S(q)/1
  phi/1 -> Fcn3/1, Fcn2/1, Fcn/1, Fcn1/1
  Fcn/1 -> Mux/1
  Fcn1/1 -> Mux/2
  Constant2/1 -> Mux/3
  Fcn2/1 -> Mux/4
  Fcn3/1 -> Mux/5
  Constant1/1 -> Mux/6

== system ddmr_for_mstc2003/direct kinematics/S*(q) matrix (3x2)/S(q) matrix (3x2)1 ==
  phi : Inport
  Constant1 : Constant
  Constant2 : Constant  Value=0
  Convert 1-D to 2-D : dspsigattribs/Convert 1-D to 2-D  M=3  N=2  frameBasedOut=off
      settings: SourceProductBaseCode=DS
  Fcn : Fcn  Expr=cos(u(3))
  Fcn1 : Fcn  Expr=sin(u(3))
  Fcn2 : Fcn  Expr=-lG*sin(u(3))
  Fcn3 : Fcn  Expr=lG*cos(u(3))
  Mux : Mux  Inputs=6
  S(q) : Outport
  wires:
  Mux/1 -> Convert 1-D to 2-D/1
  Convert 1-D to 2-D/1 -> S(q)/1
  phi/1 -> Fcn3/1, Fcn2/1, Fcn/1, Fcn1/1
  Fcn/1 -> Mux/1
  Fcn1/1 -> Mux/2
  Constant2/1 -> Mux/3
  Fcn2/1 -> Mux/4
  Fcn3/1 -> Mux/5
  Constant1/1 -> Mux/6

== system ddmr_for_mstc2003/direct kinematics/S*(q) matrix (3x2)/Subsystem ==
  Constant1 : Constant  Value=b/r
  Constant2 : Constant  Value=1/r
  Constant3 : Constant  Value=1/r
  Constant4 : Constant  Value=-b/r
  Convert 1-D to 2-D : dspsigattribs/Convert 1-D to 2-D  M=2  N=2  frameBasedOut=off
      settings: SourceProductBaseCode=DS
  Mux : Mux
  br(q) : Outport
  wires:
  Mux/1 -> Convert 1-D to 2-D/1
  Convert 1-D to 2-D/1 -> br(q)/1
  Constant2/1 -> Mux/1
  Constant3/1 -> Mux/2
  Constant1/1 -> Mux/3
  Constant4/1 -> Mux/4

== system ddmr_for_mstc2003/inverse kinematics/S*(q) matrix (3x2)/S(q) matrix (3x2)1 ==
  phi : Inport
  Constant1 : Constant
  Constant2 : Constant  Value=0
  Convert 1-D to 2-D : dspsigattribs/Convert 1-D to 2-D  M=3  N=2  frameBasedOut=off
      settings: SourceProductBaseCode=DS
  Fcn : Fcn  Expr=cos(u(3))
  Fcn1 : Fcn  Expr=sin(u(3))
  Fcn2 : Fcn  Expr=-lG*sin(u(3))
  Fcn3 : Fcn  Expr=lG*cos(u(3))
  Mux : Mux  Inputs=6
  S(q) : Outport
  wires:
  Mux/1 -> Convert 1-D to 2-D/1
  Convert 1-D to 2-D/1 -> S(q)/1
  phi/1 -> Fcn3/1, Fcn2/1, Fcn/1, Fcn1/1
  Fcn/1 -> Mux/1
  Fcn1/1 -> Mux/2
  Constant2/1 -> Mux/3
  Fcn2/1 -> Mux/4
  Fcn3/1 -> Mux/5
  Constant1/1 -> Mux/6

== system ddmr_for_mstc2003/inverse kinematics/S*(q) matrix (3x2)/Subsystem ==
  Constant1 : Constant  Value=b/r
  Constant2 : Constant  Value=1/r
  Constant3 : Constant  Value=1/r
  Constant4 : Constant  Value=-b/r
  Convert 1-D to 2-D : dspsigattribs/Convert 1-D to 2-D  M=2  N=2  frameBasedOut=off
      settings: SourceProductBaseCode=DS
  Mux : Mux
  br(q) : Outport
  wires:
  Mux/1 -> Convert 1-D to 2-D/1
  Convert 1-D to 2-D/1 -> br(q)/1
  Constant2/1 -> Mux/1
  Constant3/1 -> Mux/2
  Constant1/1 -> Mux/3
  Constant4/1 -> Mux/4
